simulink model "Cici_PV_array_RT"  (Simulink 8.5)
settings: Solver=ode3  StartTime=0.0  StopTime=10  FixedStep=20e-6  RelTol=1e-3
undefined symbols (not defined in the file): Ion, Lithium, sigbuilder_block
libraries: powerlib x9, powerlib_extras x3, rtlab x2, artemis x1, electricdrivelib x1, powerlib_meascontrol x1
settings Model: ARTEMISmethode_block_infos=$$__separator__$$V2_Cici_PV_array_RT_20us/ARTEMIS Guide$$__separator__$$  Creator=farhanm  LastModifiedBy=jiax
settings DebuggingCC: AlgebraicLoopMsg=error  SolverPrmCheckMsg=warning  FcnCallInpInsideContextMsg=UseLocalSettings

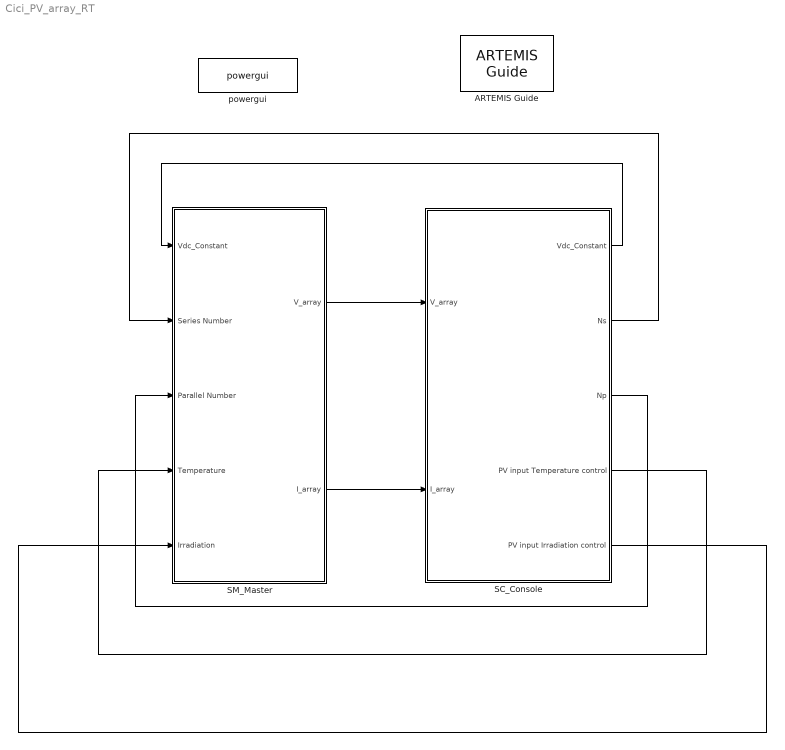
== system Cici_PV_array_RT ==
  ARTEMIS Guide : artemis/ARTEMIS/ARTEMIS Guide  Tag=FTSSmethode_opal_4hx0r99  Description=5.0_z1  lock=on  Ts=20e-6  opt=art5  dyna=off  nb_perm=4  RT_fullcomp=off  ssn=on  ssn_itvc=off  ssn_ivic=off  ssn_ext=off  ssn_solver=Art5  ssn_impulse=off  ssn_quasimpulse=off  ssn_impulse_loop=2  paraExtinctionThy=off  Thy_Impulse=on  dtc=Off  dtc_opt=normal  ao=on  simtype=off  ct_mac=off  lin_mov=off  lsp=[0.001 2]  spike_skip=Disabled  dtc_extra=1  dtc_sws=normal  dtc_pied=0.5  SPSRulesBlock=SPSRules  tre=on  ctmm=off  LF=off  dpl_type=ARTEMiS DPL  rlc_type=off  custom_type=off  para=on  ssn_ImpulseLoopBlockedStateUpdate=2  ssn_mov_iter_number=5  ssn_switch_iter_number=5  ssn_nib_type_verify=on  ssn_use_lu=on  ssn_use_ldlt=off
  SC_Console : Subsystem
  SM_Master : Subsystem
  powergui : powerlib/powergui  Priority=1  SimulationMode=Discrete  SolverType=Tustin  SampleTime=20e-6  frequency=60  SPID=off  DisableSnubberDevices=off  DisableRonSwitches=off  DisableVfSwitches=off  SwTol=0  DisplayEquations=off  Interpol=off  methode=off  Ts=100  FunctionMessages=off  echomessages=off  HookPort=off  EnableUseOfTLC=off  x0status=blocks  frequencyindice=0  Pbase=0.5e6  ErrMax=1e-4  Iterations=50  UnitsV=kV  UnitsW=MW  buscounter=0  RestoreLinks=warning  ResistiveCurrentMeasurement=off  Frange=[0:2:500]  Ylog=off  Xlog=on  ShowGrid=off  save=off  variable=ZData  structure=0  ZoomFFT=off  StartTime=0.0  cycles=1  DisplayStyle=1  fundamental=60  FreqAxis=off  MaxFrequency=1000  frequencyindicesteady=1  RmsSteady=1  display=off
  wires:
  SM_Master/1(V_array) -> SC_Console/1(V_array)
  SM_Master/2(I_array) -> SC_Console/2(I_array)
  SC_Console/1(" Vdc_Constant") -> SM_Master/1(Vdc_Constant)
  SC_Console/2(" Ns") -> SM_Master/2(Series Number)
  SC_Console/3(" Np") -> SM_Master/3(Parallel Number)
  SC_Console/4(" PV input Temperature control") -> SM_Master/4(Temperature)
  SC_Console/5(PV input Irradiation control) -> SM_Master/5(Irradiation)

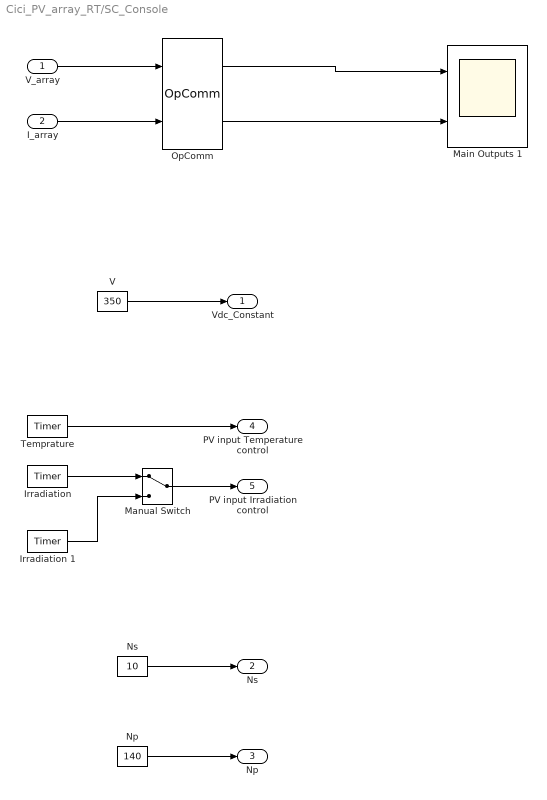
== system Cici_PV_array_RT/SC_Console ==
  V_array : Inport
  I_array : Inport  Port=2
  "Irradiation " : powerlib_extras/Control  Blocks/Timer  t=[0 10 35]  e=[1000 500 1000]
  Irradiation 1 : powerlib_extras/Control  Blocks/Timer  t=[0 10 15 20 25 30 35 40 45 50 55]  e=[1000 1000 950 800 900 700 650 600 600 500 450]
  Main Outputs 1 : Scope  NumInputPorts=2
      settings: TimeRange=10  YMin=0~375  YMax=900~700  SaveName=ScopeData24
  Manual Switch : ManualSwitch
  Np : Constant  Value=140
  Ns : Constant  Value=10
  OpComm : rtlab/OpComm  nbport=2  groupe_acq=1  subsys_rate=20e-6  st=0  Synchronization=on  Interpolation=on  Threshold=1.0  Missed_Data=off  Sim_Time=off  Samples=off  dynSigOut=off  from_console=0  warning_done=off  writeOpCommFile=off  Offset=off
  Temprature : powerlib_extras/Control  Blocks/Timer  t=[0 40 45]  e=[25 25 25]
  V : Constant  Value=350
  " Vdc_Constant" : Outport
  " Ns" : Outport  Port=2
  " Np" : Outport  Port=3
  " PV input Temperature control" : Outport  Port=4
  PV input Irradiation control : Outport  Port=5
  wires:
  V/1 -> " Vdc_Constant"/1
  Ns/1 -> " Ns"/1
  Temprature/1 -> " PV input Temperature control"/1
  Np/1 -> " Np"/1
  "Irradiation "/1 -> Manual Switch/1
  Irradiation 1/1 -> Manual Switch/2
  Manual Switch/1 -> PV input Irradiation control/1
  V_array/1 -> OpComm/1
  I_array/1 -> OpComm/2
  OpComm/1 -> Main Outputs 1/1
  OpComm/2 -> Main Outputs 1/2

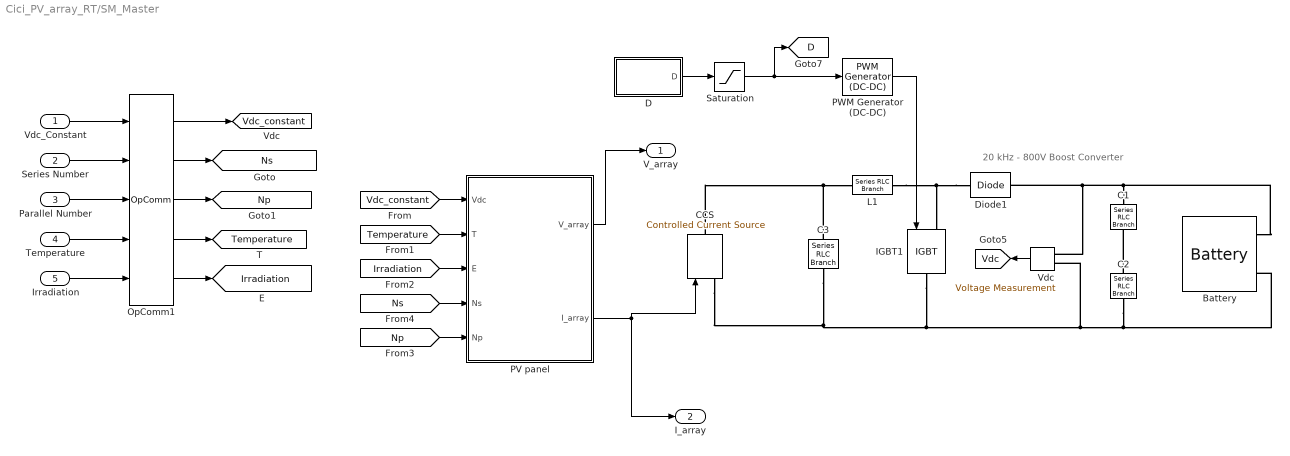
== system Cici_PV_array_RT/SM_Master ==
  note: 20 kHz - 800V
      | Boost Converter
  Vdc_Constant : Inport
  Series Number : Inport  Port=2
  Parallel Number : Inport  Port=3
  Temperature : Inport  Port=4
  Irradiation : Inport  Port=5
  Battery : electricdrivelib/Extra Sources/Battery  BatType=Lithium-Ion  ShowDetailedParameters=off  NomV=800  NomQ=1000  SOC=10  PresetModel=on  MaxQ=1000  FullV=931.1897  Dis_rate=434.7826  R=0.008  Normal_OP=904.3478  expZone="[864.3087      49.13043]"  current=[6.5 13 32.5]  Units=Time  Batt_Tr=30
  C1 : powerlib/Elements/Series RLC Branch  LConnTagsString=__new0  RConnTagsString=__new0  BranchType=C  Resistance=1.0  Inductance=1.0  SetiL0=off  InitialCurrent=0  Capacitance=12000e-06  Setx0=off  InitialVoltage=0  Measurements=None
  C2 : powerlib/Elements/Series RLC Branch  LConnTagsString=__new0  RConnTagsString=__new0  BranchType=C  Resistance=1.0  Inductance=1.0  SetiL0=off  InitialCurrent=0  Capacitance=12000e-06  Setx0=off  InitialVoltage=0  Measurements=None
  C3 : powerlib/Elements/Series RLC Branch  LConnTagsString=__new0  RConnTagsString=__new0  BranchType=C  Resistance=1.0  Inductance=1.0  SetiL0=off  InitialCurrent=0  Capacitance=100e-6  Setx0=off  InitialVoltage=0  Measurements=Branch voltage
  CCS : powerlib/Electrical Sources/Controlled Current Source  Initialize=on  Source_Type=DC  Amplitude=0  Phase=0  Frequency=0  Measurements=Current
  D : Subsystem  Tag=STV Subsys  LoadFcn=sigbuilder_block('load');  StartFcn=sigbuilder_block('start');  StopFcn=sigbuilder_block('stop');  ClipboardFcn=sigbuilder_block('clipboard');  mask(Sigbuilder block){}
      mask help: Sigbuilder GUI
      mask init:
      | if ~strcmp(get_param(bdroot(gcbh),'SimulationStatus'),'stopped') tuvar = sigbuilder_block('maskInit'); end
      settings: CopyFcn=sigbuilder_block('copy');  DeleteFcn=sigbuilder_block('delete');  ModelCloseFcn=sigbuilder_block('modelClose');  PreSaveFcn=sigbuilder_block('preSave');  PauseFcn=sigbuilder_block('pause')  ContinueFcn=sigbuilder_block('continue')  NameChangeFcn=sigbuilder_block('namechange');  OpenFcn=sigbuilder_block('open',[6 30 1012.5 446.25 ]);  CloseFcn=sigbuilder_block('close');
      mask Display: plot(0,0,100,100,[10,10,40,40,10],[80,20,20,80,80],[40,10],[50,50], [40,27,10],[65,72,56],[40,25,25,10],[28,28,43,43]);
  Diode1 : powerlib/Power Electronics/Diode  Ron=1e-4  Lon=0  Vf=0  IC=0  UseSnubber=off  Rs=inf  Cs=inf  Measurements=off
  IGBT1 : powerlib/Power Electronics/IGBT  Ron=0.001  Lon=0  Vf=0  Tf=0  Tt=0  IC=0  Rs=1e5  Cs=inf  Measurements=off
  L1 : powerlib/Elements/Series RLC Branch  LConnTagsString=__new0  RConnTagsString=__new0  BranchType=RL  Resistance=0.005  Inductance=5e-3  SetiL0=off  InitialCurrent=0  Capacitance=1e-6  Setx0=off  InitialVoltage=0  Measurements=None
  OpComm1 : rtlab/OpComm  nbport=5  groupe_acq=1  subsys_rate=20e-6  st=0  Synchronization=on  Interpolation=on  Threshold=1.0  Missed_Data=off  Sim_Time=off  Samples=off  dynSigOut=off  from_console=1  warning_done=off  writeOpCommFile=off  Offset=off
  "PV panel " : Subsystem  mask{Voc=43.8, Isc=5, Vmpp=35, Impp=4.58, beta_Voc=-0.1, alpha_Isc=0.00002, Ncell=40}
      mask prompts: Voc "Open Circuit Voltage Voc (V)"; Isc "Short Circuit Current Isc (A)"; Vmpp "Voltage at Maximum Power Point Vmpp (V)"; Impp "Current at Maximum Power Point Impp (A)"; beta_Voc "Temperature Coefficient of Voc (%/deg.C)"; alpha_Isc "Temperature Coefficient of Isc (%/deg.C)"; Ncell "Cells per Module (Ncell)"
  PWM Generator (DC-DC) : powerlib_meascontrol/Pulse & Signal Generators/PWM Generator (DC-DC)  Fsw=20000  Ts=20e-06
  Saturation : Saturate  UpperLimit=0.8  LowerLimit=0.2
  "Vdc " : powerlib/Measurements/Voltage Measurement  Tag=PoWeRsYsTeMmEaSuReMeNt  PhasorSimulation=off  OutputType=Magnitude  PSBequivalent=0
  V_array : Outport
  I_array : Outport  Port=2
  tag scope: D=global, Irradiation=global, Np=global, Ns=global, Temperature=global, Vdc=global, Vdc_constant=global
  wires:
  "Vdc "/1 -> [Vdc]
  Saturation/1 -> PWM Generator (DC-DC)/1, [D]
  D/1(D) -> Saturation/1
  PWM Generator (DC-DC)/1 -> IGBT1/1
  Vdc_Constant/1 -> OpComm1/1
  Series Number/1 -> OpComm1/2
  Parallel Number/1 -> OpComm1/3
  Temperature/1 -> OpComm1/4
  Irradiation/1 -> OpComm1/5
  OpComm1/1 -> [Vdc_constant]
  OpComm1/2 -> [Ns]
  OpComm1/3 -> [Np]
  OpComm1/4 -> [Temperature]
  OpComm1/5 -> [Irradiation]
  [Temperature] -> "PV panel "/2(T)
  [Irradiation] -> "PV panel "/3(E)
  [Vdc_constant] -> "PV panel "/1(Vdc)
  "PV panel "/1(V_array) -> V_array/1
  "PV panel "/2(I_array) -> CCS/1, I_array/1
  [Ns] -> "PV panel "/4(Ns)
  [Np] -> "PV panel "/5(Np)
  connections:
  "Vdc "/LConn1 -- Battery/LConn1 -- C1/LConn1 -- Diode1/RConn1
  Diode1/LConn1 -- IGBT1/LConn1 -- L1/RConn1
  "Vdc "/LConn2 -- CCS/LConn1 -- C3/RConn1 -- IGBT1/RConn1 -- C2/RConn1 -- Battery/LConn2
  C3/LConn1 -- L1/LConn1 -- CCS/RConn1
  C2/LConn1 -- C1/RConn1

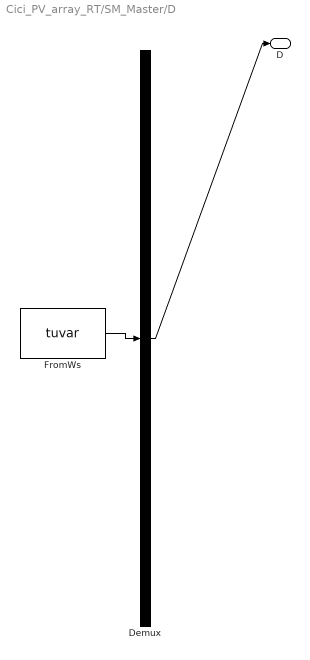
== system Cici_PV_array_RT/SM_Master/D ==
  Demux : Demux  Tag=STV Demux  Outputs=1
  FromWs : FromWorkspace  Tag=STV FromWs  VariableName=tuvar  SampleTime=0  SigBuilderData=DataTag0  VnvData=DataTag1
      SigBuilderData=|
      | common.afterFinalStr = 'Extrapolate'
      | common.sampleTime = '0'
      | dataSet(1).timeRange = [0 2]
      | dataSet(1).name = 'Constant Irradiance'
      | dataSet(2).timeRange = [0 2]
      | dataSet(2).name = 'Step Irradiance'
      | dataSet(3).timeRange = [0 3]
      | dataSet(3).name = 'Ramp-up/down Irradiance'
      | sbobj.Groups(1).Name = 'Constant Irradiance'
      | sbobj.Groups(1).Signals.Name = 'D'
      | sbobj.Groups(1).Signals.XData = [0 1.2 1.2 1.8 1.8 3]
      | sbobj.Groups(1).Signals.YData = [0 0 1 1 0 0]
      | sbobj.Groups(1).TimeRange = [0 3]
      | sbobj.Groups(2).Name = 'Step Irradiance'
      | sbobj.Groups(2).Signals.Name = 'D'
      | sbobj.Groups(2).Signals.XData = [0 1.2 1.2 1.8 1.8 3]
      | sbobj.Groups(2).Signals.YData = [0 0 1 1 0 0]
      | sbobj.Groups(2).TimeRange = [0 3]
      | sbobj.Groups(3).Name = 'Ramp-up/down Irradiance'
      | sbobj.Groups(3).Signals.Name = 'D'
      | sbobj.Groups(3).Signals.XData = [0 0.4 0.699 0.699 0.8 0.8 3]
      | sbobj.Groups(3).Signals.YData = [0.4 0.4 0.601 0.598 0.599 0.4995 0.4995]
      | sbobj.Groups(3).TimeRange = [0 3]
  D : Outport  Tag=STV Outport
  wires:
  FromWs/1 -> Demux/1
  Demux/1 -> D/1

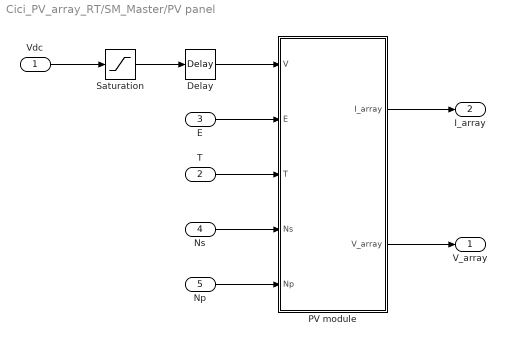
== system Cici_PV_array_RT/SM_Master/PV panel  ==
  Vdc : Inport
  T : Inport  Port=2
  E : Inport  Port=3
  Ns : Inport  Port=4
  Np : Inport  Port=5
  Delay : TransportDelay  DelayTime=0.05
  PV module : Subsystem
  Saturation : Saturate  UpperLimit=876  LowerLimit=0
  V_array : Outport
  I_array : Outport  Port=2
  wires:
  Saturation/1 -> Delay/1
  E/1 -> PV module/2(E)
  T/1 -> PV module/3(T)
  Vdc/1 -> Saturation/1
  Delay/1 -> PV module/1(V)
  Ns/1 -> PV module/4(Ns)
  Np/1 -> PV module/5(Np)
  PV module/1(I_array) -> I_array/1
  PV module/2(V_array) -> V_array/1

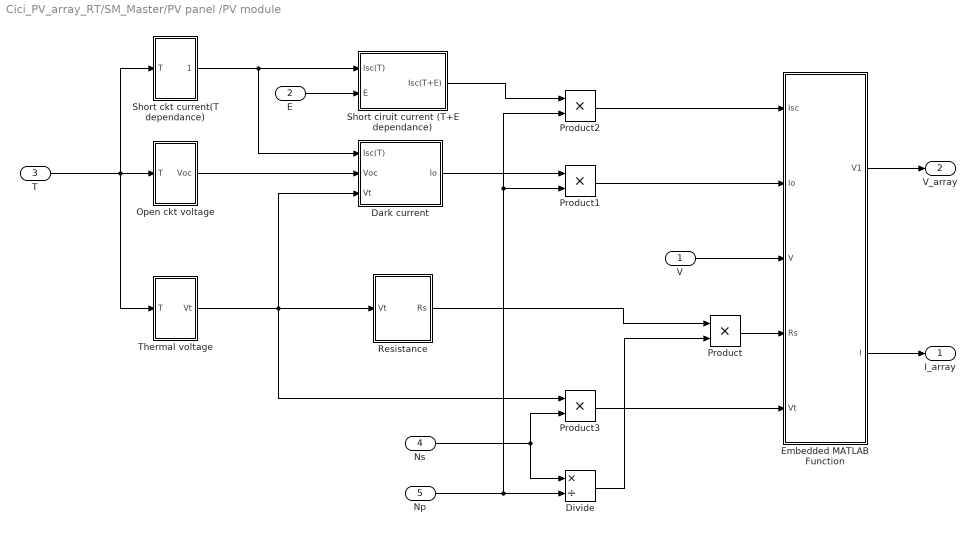
== system Cici_PV_array_RT/SM_Master/PV panel /PV module ==
  V : Inport
  E : Inport  Port=2
  T : Inport  Port=3
  Ns : Inport  Port=4
  Np : Inport  Port=5
  Dark current : Subsystem
  Divide : Product  Inputs=*/
  Embedded MATLAB Function : MATLAB Function  TreatAsAtomicUnit=on
  Open ckt voltage : Subsystem
  Product{,1..3} (4 alike) : Product
  Resistance : Subsystem
  Short ciruit current (T+E dependance) : Subsystem
  "Short ckt current(T dependance) " : Subsystem
  Thermal voltage : Subsystem
  I_array : Outport
  V_array : Outport  Port=2
  wires:
  Thermal voltage/1(Vt) -> Product3/1, Resistance/1(Vt), Dark current/3(Vt)
  T/1 -> "Short ckt current(T dependance) "/1(T), Thermal voltage/1(T), Open ckt voltage/1(T)
  E/1 -> Short ciruit current (T+E dependance)/2(E)
  Open ckt voltage/1(Voc) -> Dark current/2(Voc)
  Embedded MATLAB Function/2(I) -> I_array/1
  Embedded MATLAB Function/1(V1) -> V_array/1
  V/1 -> Embedded MATLAB Function/3(V)
  Ns/1 -> Product3/2, Divide/1
  Np/1 -> Divide/2, Product1/2, Product2/2
  Product/1 -> Embedded MATLAB Function/4(Rs)
  Product1/1 -> Embedded MATLAB Function/2(Io)
  Product2/1 -> Embedded MATLAB Function/1(Isc)
  Product3/1 -> Embedded MATLAB Function/5(Vt)
  Dark current/1(Io) -> Product1/1
  Resistance/1(Rs) -> Product/1
  Divide/1 -> Product/2
  "Short ckt current(T dependance) "/1(Isc(T)) -> Dark current/1(Isc(T)), Short ciruit current (T+E dependance)/1(Isc(T))
  Short ciruit current (T+E dependance)/1(Isc(T+E)) -> Product2/1

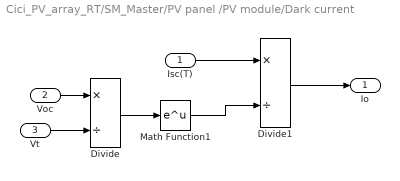
== system Cici_PV_array_RT/SM_Master/PV panel /PV module/Dark current ==
  Isc(T) : Inport
  Voc : Inport  Port=2
  Vt : Inport  Port=3
  Divide : Product  Inputs=*/
  Divide1 : Product  Inputs=*/
  Math Function1 : Math  SaturateOnIntegerOverflow=on
  Io : Outport
  wires:
  Divide/1 -> Math Function1/1
  Math Function1/1 -> Divide1/2
  Vt/1 -> Divide/2
  Voc/1 -> Divide/1
  Isc(T)/1 -> Divide1/1
  Divide1/1 -> Io/1

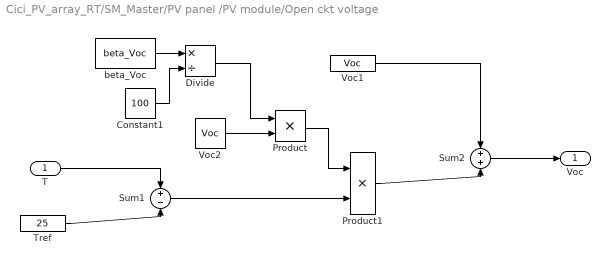
== system Cici_PV_array_RT/SM_Master/PV panel /PV module/Open ckt voltage ==
  T : Inport
  Constant1 : Constant  Value=100
  Divide : Product  Inputs=*/
  Product : Product
  Product1 : Product  RndMeth=Zero
  Sum1 : Sum  Inputs=+-
  Sum2 : Sum
  Tref : Constant  Value=25
  Voc1 : Constant  Value=Voc
  Voc2 : Constant  Value=Voc
  beta_Voc : Constant  Value=beta_Voc
  Voc : Outport
  wires:
  Tref/1 -> Sum1/2
  T/1 -> Sum1/1
  Sum1/1 -> Product1/2
  Voc1/1 -> Sum2/1
  Product1/1 -> Sum2/2
  Sum2/1 -> Voc/1
  beta_Voc/1 -> Divide/1
  Constant1/1 -> Divide/2
  Divide/1 -> Product/1
  Voc2/1 -> Product/2
  Product/1 -> Product1/1

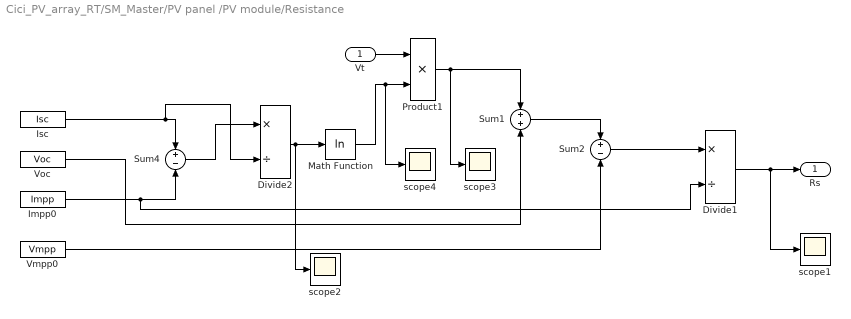
== system Cici_PV_array_RT/SM_Master/PV panel /PV module/Resistance ==
  Vt : Inport
  Divide1 : Product  Inputs=*/
  Divide2 : Product  Inputs=*/
  Impp0 : Constant  Value=Impp
  Isc : Constant  Value=Isc
  Math Function : Math  Operator=log  SaturateOnIntegerOverflow=on
  Product1 : Product  RndMeth=Zero
  Sum1 : Sum
  Sum2 : Sum  Inputs=+-
  Sum4 : Sum  Inputs=+-
  Vmpp0 : Constant  Value=Vmpp
  Voc : Constant  Value=Voc
  scope{1..4} (4 alike) : Scope
      scope1 settings: SaveName=ScopeData10
      scope2 settings: SaveName=ScopeData11
      scope3 settings: SaveName=ScopeData12
      scope4 settings: SaveName=ScopeData13
  Rs : Outport
  wires:
  Isc/1 -> Sum4/1, Divide2/2
  Impp0/1 -> Sum4/2, Divide1/2
  Divide2/1 -> Math Function/1, scope2/1
  Voc/1 -> Sum1/2
  Product1/1 -> Sum1/1, scope3/1
  Sum1/1 -> Sum2/1
  Vmpp0/1 -> Sum2/2
  Sum2/1 -> Divide1/1
  Divide1/1 -> Rs/1, scope1/1
  Vt/1 -> Product1/1
  Sum4/1 -> Divide2/1
  Math Function/1 -> Product1/2, scope4/1

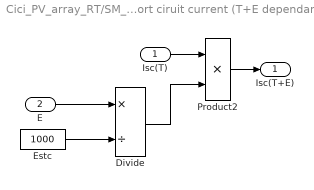
== system Cici_PV_array_RT/SM_Master/PV panel /PV module/Short ciruit current (T+E dependance) ==
  Isc(T) : Inport
  E : Inport  Port=2
  Divide : Product  Inputs=*/
  Estc : Constant  Value=1000
  Product2 : Product  RndMeth=Zero
  Isc(T+E) : Outport
  wires:
  E/1 -> Divide/1
  Estc/1 -> Divide/2
  Divide/1 -> Product2/2
  Product2/1 -> Isc(T+E)/1
  Isc(T)/1 -> Product2/1

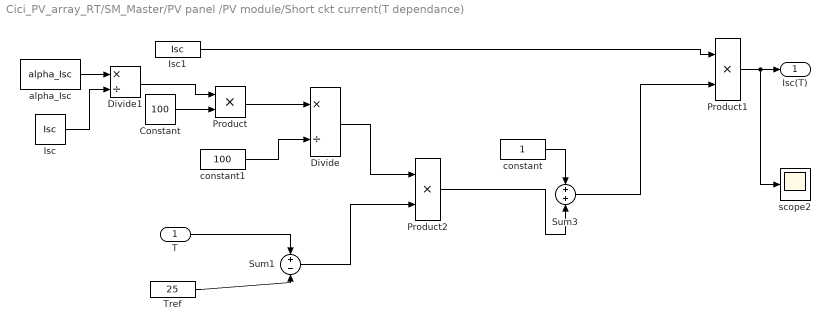
== system Cici_PV_array_RT/SM_Master/PV panel /PV module/Short ckt current(T dependance)  ==
  T : Inport
  Constant : Constant  Value=100
  Divide : Product  Inputs=*/
  Divide1 : Product  Inputs=*/
  Isc : Constant  Value=Isc
  Isc1 : Constant  Value=Isc
  Product : Product
  Product1 : Product  RndMeth=Zero
  Product2 : Product  RndMeth=Zero
  Sum1 : Sum  Inputs=+-
  Sum3 : Sum
  Tref : Constant  Value=25
  alpha_Isc : Constant  Value=alpha_Isc
  constant : Constant
  constant1 : Constant  Value=100
  scope2 : Scope
      settings: SaveName=ScopeData16
  Isc(T) : Outport
  wires:
  Isc1/1 -> Product1/1
  constant1/1 -> Divide/2
  T/1 -> Sum1/1
  Tref/1 -> Sum1/2
  Product1/1 -> Isc(T)/1, scope2/1
  Divide/1 -> Product2/1
  Sum1/1 -> Product2/2
  constant/1 -> Sum3/1
  Product2/1 -> Sum3/2
  Sum3/1 -> Product1/2
  alpha_Isc/1 -> Divide1/1
  Isc/1 -> Divide1/2
  Divide1/1 -> Product/1
  Constant/1 -> Product/2
  Product/1 -> Divide/1

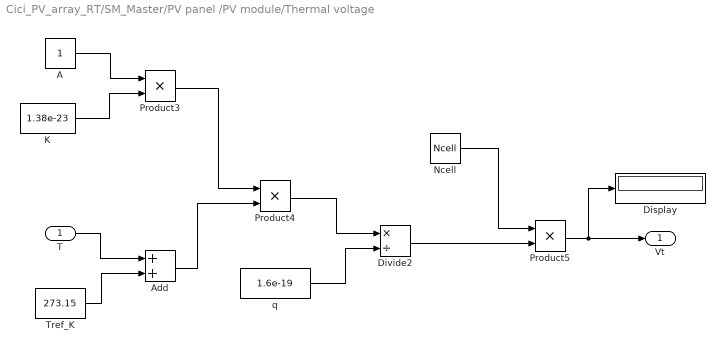
== system Cici_PV_array_RT/SM_Master/PV panel /PV module/Thermal voltage ==
  T : Inport
  A : Constant
  Add : Sum
  Display : Display
  Divide2 : Product  Inputs=*/
  K : Constant  Value=1.38e-23
  Ncell : Constant  Value=Ncell
  Product3 : Product
  Product4 : Product
  Product5 : Product
  Tref_K : Constant  Value=273.15
  q : Constant  Value=1.6e-19
  Vt : Outport
  wires:
  T/1 -> Add/1
  Tref_K/1 -> Add/2
  A/1 -> Product3/1
  K/1 -> Product3/2
  Product3/1 -> Product4/1
  Add/1 -> Product4/2
  Product4/1 -> Divide2/1
  q/1 -> Divide2/2
  Product5/1 -> Display/1, Vt/1
  Ncell/1 -> Product5/1
  Divide2/1 -> Product5/2

== matlab function SM_Master/PV panel /PV module/Embedded MATLAB Function ==
  data: Isc input double; V1 output double; Io input double; I output double; V input double; Rs input double; Vt input double
function [V1,I] = fcn(Isc, Io,V,Rs,Vt)
 
 %% Newton Raphson Method used in power factory
Istart=0.01;
FI0=0; 
FpI0=0; 
I1=Istart; 

FI1=0; 
FpI1=0; 
I2=I1; 

FI2=0; 
FpI2=0; 
I3=I2; 

FI3=0; 
FpI3=0; 
I4=4.58;
 
 
FI0=Istart-Isc+Io*(exp((V+Istart*Rs)/Vt)-1);
FpI0=1+Io*(exp((V+Istart*Rs)/Vt))*Rs/Vt;
I1=Istart-FI0/FpI0;

FI1=I1-Isc+Io*(exp((V+I1*Rs)/Vt)-1);
FpI1=1+Io*(exp((V+I1*Rs)/Vt))*Rs/Vt;
I2=I1-FI1/FpI1;

FI2=I2-Isc+Io*(exp((V+I2*Rs)/Vt)-1);
FpI2=1+Io*(exp((V+I2*Rs)/Vt))*Rs/Vt;
I3=I2-FI2/FpI2;

FI3=I3-Isc+Io*(exp((V+I3*Rs)/Vt)-1);
FpI3=1+Io*(exp((V+I3*Rs)/Vt))*Rs/Vt;
I4=I3-FI3/FpI3;
I=I4
V1=V;
